simulink model "A14_Servoachse_Kaskade"  (R2017b)
settings: Solver=ode45  StartTime=0.0  StopTime=10  FixedStep=0.001  MaxStep=1e-4  RelTol=1e-3  EnableMultiTasking=on
values from neighbouring files (symbols this model uses):
  CD = 1e1    (= 10)    [A14_Konstanten.m]    (also in A17_Konstanten.m = 100; A8_Konstanten.m = 20; A9_Konstanten.m = 0.1)
  CF = 1e4    (= 10000)    [A13_Konstanten.m]    (also in A14_Konstanten.m; A17_Konstanten.m = 50000; A8_Konstanten.m = 10000000; A9_Konstanten.m)
  CM = 7.1e-7    (= 7.1e-07)    [A10_Konstanten.m]    (also in A13_Konstanten.m; A14_Konstanten.m; A16_Konstanten.m)
  CR = 0.2    [A13_Konstanten.m]    (also in A14_Konstanten.m; A17_Konstanten.m = 100; A9_Konstanten.m = 1; Z_Parametrisierung_Skript.m = [0.5,1,5])
  FReib = 0.5    [A13_Konstanten.m]    (also in A14_Konstanten.m)
  Imax = 4.81    [A10_Konstanten.m]    (also in A13_Konstanten.m; A14_Konstanten.m; A16_Konstanten.m)
  JM = JR + JG    (= 1.38e-06)    [A13_Konstanten.m]    (also in A14_Konstanten.m)
  KM = 38.4e-3    (= 0.0384)    [A10_Konstanten.m]    (also in A13_Konstanten.m; A14_Konstanten.m; A16_Konstanten.m)
  KN = 1/(2*pi*KM)    (= 4.14465997635)    [A10_Konstanten.m]    (also in A13_Konstanten.m; A14_Konstanten.m; A16_Konstanten.m)
  LA = 4.64e-4    (= 0.000464)    [A10_Konstanten.m]    (also in A13_Konstanten.m; A14_Konstanten.m; A16_Konstanten.m)
  m1 = 1    [A13_Konstanten.m]    (also in A14_Konstanten.m; A17_Konstanten.m = 4; A8_Konstanten.m = 20)
  nmax = 99    [A10_Konstanten.m]    (also in A13_Konstanten.m; A14_Konstanten.m; A16_Konstanten.m)
  R = 0.02    [A10_Konstanten.m]    (also in A13_Konstanten.m = 0.04; A14_Konstanten.m = 0.04; A16_Konstanten.m)
  RA = 4.99    [A10_Konstanten.m]    (also in A13_Konstanten.m; A14_Konstanten.m; A16_Konstanten.m)
  Ti = Ue/(2*pi*R)    (= 15.9154943092)    [A14_Konstanten.m]
  Tisens = 2e-5    (= 2e-05)    [A14_Konstanten.m]
  Tnsens = 8e-5    (= 8e-05)    [A14_Konstanten.m]
  TPWM = 2e-5    (= 2e-05)    [A14_Konstanten.m]
  Tssens = Tnsens    (= 8e-05)    [A14_Konstanten.m]
  TVn = 4*(2*(TPWM+Tisens)+Tnsens)    (= 0.00064)    [A14_Konstanten.m]
  Ue = 4    [A13_Konstanten.m]    (also in A14_Konstanten.m)
  Umax = 24    [A10_Konstanten.m]    (also in A13_Konstanten.m; A14_Konstanten.m; A16_Konstanten.m; A17_Konstanten.m = 120)
  WGrad = 0.85    [A13_Konstanten.m]    (also in A14_Konstanten.m)
undefined symbols (not defined in the file or in its folder): sigbuilder_block
libraries: simulink x4
settings Model: Creator=jbaur  LastModifiedBy=jbaur
settings DataIOCC: ExternalInput=X1  SaveFormat=StructureWithTime  InspectSignalLogs=on  SignalLoggingName=sigsOut
settings OptimizationCC: DefaultParameterBehavior=Inlined  InlineInvariantSignals=on  BufferReuse=off  ExpressionDepthLimit=2147483647  InitFltsAndDblsToZero=on  LifeSpan=inf
settings DebuggingCC: SaveWithParameterizedLinksMsg=none  SignalResolutionControl=TryResolveAllWithWarning  MultiTaskDSMMsg=warning  MultiTaskCondExecSysMsg=none  StateNameClashWarn=warning  InitInArrayFormatMsg=none  SFUnexpectedBacktrackingDiag=warning  SFNoUnconditionalDefaultTransitionDiag=warning  SFExecutionAtInitializationDiag=none
settings HardwareCC: ProdBitPerPointer=32  ProdBitPerSizeT=32  ProdBitPerPtrDiffT=32  ProdLargestAtomicFloat=None  ProdIntDivRoundTo=Undefined  ProdEndianess=Unspecified  ProdWordSize=32  ProdHWDeviceType=32-bit Generic  TargetBitPerPointer=64  TargetBitPerSizeT=64  TargetBitPerPtrDiffT=64  TargetLongLongMode=on  TargetIntDivRoundTo=Zero  TargetEndianess=LittleEndian  TargetWordSize=64  TargetHWDeviceType=MATLAB Host  ProdEqTarget=off
settings ModelReferenceCC: PropagateSignalLabelsOutOfModel=off
settings CodeAppCC: StateflowObjectComments=on
settings GRTTargetCC: TargetFcnLib=ansi_tfl_tmw.mat  TargetLangStandard=C89/C90 (ANSI)  ModelReferenceCompliant=off  GeneratePreprocessorConditionals=Disable all  CombineOutputUpdateFcns=off  MatFileLogging=off  GRTInterface=on
settings ConfigComp: CovMetricSettings=dw  CovHtmlReporting=on  CovSaveCumulativeToWorkspaceVar=on  CovSaveSingleToWorkspaceVar=on  CovExternalEMLEnable=off  CovSFcnEnable=off

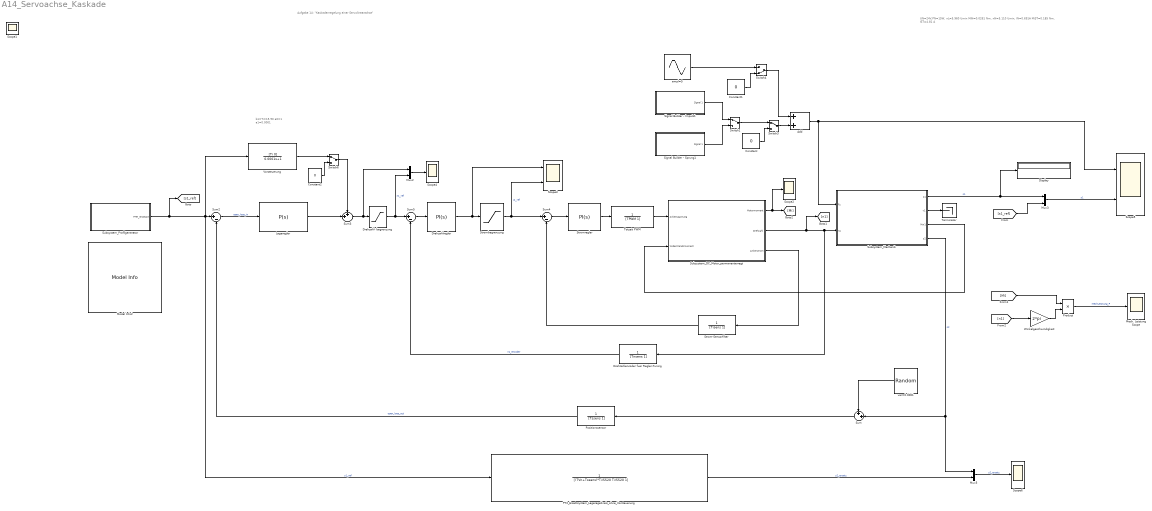
== system A14_Servoachse_Kaskade ==
  note: b1=Ti=15.90
      | a0=1
      | a1=0.0001
  note: Aufgabe 14: "Kaskadenregelung einer Servolinearachse"
  note: UN=24V,PN=15W, nL=5.960 Umin
      | MiN=0.0261 Nm, nN=5.110 Umin, IN=0.691A
      | MiST=0.185 Nm, IST=4.81 A
  Add : Sum
  Constant : Constant  Value=0
  Constant1 : Constant  Value=0
  Constant2 : Constant  Value=0
  Display : Display
  Drehzahl- begrenzung : Saturate  UpperLimit=nmax  LowerLimit=-nmax
  Drehzahlencoder fuer Regler-Tuning : TransferFcn  Denominator=[Tnsens 1]
  Drehzahlregler : simulink/Continuous/PID Controller  Controller=PI  TimeDomain=Continuous-time  SampleTime=-1  IntegratorMethod=Forward Euler  FilterMethod=Forward Euler  Form=Ideal  UseFilter=on  ControllerParametersSource=internal  P=1  I=1  D=0  N=1000  InitialConditionSource=internal  InitialConditionForIntegrator=0  InitialConditionForFilter=0  ExternalReset=none  LimitOutput=on  UpperSaturationLimit=Imax  LowerSaturationLimit=-Imax  LinearizeAsGain=off  AntiWindupMode=clamping  Kb=1  TrackingMode=off  Kt=1  PParamMin=[]  PParamMax=[]  IParamMin=[]  IParamMax=[]  DParamMin=[]  DParamMax=[]  NParamMin=[]  NParamMax=[]  KbParamMin=[]  KbParamMax=[]  KtParamMin=[]  KtParamMax=[]  POutMin=[]  POutMax=[]  IOutMin=[]  IOutMax=[]  DOutMin=[]  DOutMax=[]  NOutMin=[]  NOutMax=[]  KbOutMin=[]  KbOutMax=[]  KtOutMin=[]  KtOutMax=[]  IntegratorOutMin=[]  IntegratorOutMax=[]  FilterOutMin=[]  FilterOutMax=[]  SumOutMin=[]  SumOutMax=[]  SumI1OutMin=[]  SumI1OutMax=[]  SumI2OutMin=[]  SumI2OutMax=[]  SumI3OutMin=[]  SumI3OutMax=[]  SumDOutMin=[]  SumDOutMax=[]  SaturationOutMin=[]  SaturationOutMax=[]  IntegratorContinuousStateAttributes=''  IntegratorStateMustResolveToSignalObject=off  IntegratorRTWStateStorageClass=Auto  FilterContinuousStateAttributes=''  FilterStateMustResolveToSignalObject=off  FilterRTWStateStorageClass=Auto  DifferentiatorICPrevScaledInput=0  DifferentiatorOutMin=[]  DifferentiatorOutMax=[]  InitialConditionSetting=State (most efficient)  FilterDiffOutCoefMin=[]  FilterDiffOutCoefMax=[]  SumDenOutMin=[]  SumDenOutMax=[]  SumNumOutMin=[]  SumNumOutMax=[]  ReciprocalOutMin=[]  ReciprocalOutMax=[]  DivideOutMin=[]  DivideOutMax=[]  TunerSelectOption=Transfer Function Based (PID Tuner App)
  Lageregler : simulink/Continuous/PID Controller  Controller=P  TimeDomain=Continuous-time  SampleTime=-1  IntegratorMethod=Forward Euler  FilterMethod=Forward Euler  Form=Ideal  UseFilter=on  ControllerParametersSource=internal  P=1  I=2096.01243911413  D=0  N=100  InitialConditionSource=internal  InitialConditionForIntegrator=0  InitialConditionForFilter=0  ExternalReset=none  LimitOutput=off  UpperSaturationLimit=nmax  LowerSaturationLimit=-nmax  LinearizeAsGain=off  AntiWindupMode=none  Kb=1  TrackingMode=off  Kt=1  PParamMin=[]  PParamMax=[]  IParamMin=[]  IParamMax=[]  DParamMin=[]  DParamMax=[]  NParamMin=[]  NParamMax=[]  KbParamMin=[]  KbParamMax=[]  KtParamMin=[]  KtParamMax=[]  POutMin=[]  POutMax=[]  IOutMin=[]  IOutMax=[]  DOutMin=[]  DOutMax=[]  NOutMin=[]  NOutMax=[]  KbOutMin=[]  KbOutMax=[]  KtOutMin=[]  KtOutMax=[]  IntegratorOutMin=[]  IntegratorOutMax=[]  FilterOutMin=[]  FilterOutMax=[]  SumOutMin=[]  SumOutMax=[]  SumI1OutMin=[]  SumI1OutMax=[]  SumI2OutMin=[]  SumI2OutMax=[]  SumI3OutMin=[]  SumI3OutMax=[]  SumDOutMin=[]  SumDOutMax=[]  SaturationOutMin=[]  SaturationOutMax=[]  IntegratorContinuousStateAttributes=''  IntegratorStateMustResolveToSignalObject=off  IntegratorRTWStateStorageClass=Auto  FilterContinuousStateAttributes=''  FilterStateMustResolveToSignalObject=off  FilterRTWStateStorageClass=Auto  DifferentiatorICPrevScaledInput=0  DifferentiatorOutMin=[]  DifferentiatorOutMax=[]  InitialConditionSetting=State (most efficient)  FilterDiffOutCoefMin=[]  FilterDiffOutCoefMax=[]  SumDenOutMin=[]  SumDenOutMax=[]  SumNumOutMin=[]  SumNumOutMax=[]  ReciprocalOutMin=[]  ReciprocalOutMax=[]  DivideOutMin=[]  DivideOutMax=[]  TunerSelectOption=Transfer Function Based (PID Tuner App)
  Mech. Leistung Scope : Scope
  Model Info2 : simulink/Model-Wide Utilities/Model Info  Frame=on  DisplayStringWithTags=|  HorizontalTextAlignment=Left  LeftAlignmentValue=0.02
      | Bewegungsprofil:
      | ------------------------
      | Tmax = 1s
      | smax = 0,5m
      | vmax = 1 m/s
      | amax = 2 m/s^2
  Mux2 : Mux  Inputs=2
  Mux3 : Mux  Inputs=2
  Mux5 : Mux  Inputs=2
  PT2_Ersatzsystem_Lageregelkreis_ohne_Vorsteuerung : TransferFcn  Denominator=[(TVn+Tssens)*Ti/5520 Ti/5520 1]
  "Positionssensor " : TransferFcn  Denominator=[Tssens 1]
  Product : Product  RndMeth=Zero
  Scope{1..2,4,6} (4 alike) : Scope
  Scope3 : Scope  NumInputPorts=2
  Scope5 : Scope  NumInputPorts=2
  Signal Builder - Impuls1 : Subsystem  Tag=STV Subsys  LoadFcn=sigbuilder_block('load');  StartFcn=sigbuilder_block('start');  StopFcn=sigbuilder_block('stop');  ClipboardFcn=sigbuilder_block('clipboard');  mask(Sigbuilder block){tuvar=[0:10]}
      mask help: Simulink:masks:SigbuilderBlock_MD
      mask init:
      | if ~strcmp(get_param(bdroot(gcbh),'SimulationStatus'),'stopped') tuvar = sigbuilder_block('maskInit'); end
      settings: CopyFcn=sigbuilder_block('copy');  DeleteFcn=sigbuilder_block('delete');  ModelCloseFcn=sigbuilder_block('modelClose');  PreSaveFcn=sigbuilder_block('preSave');  PauseFcn=sigbuilder_block('pause');  ContinueFcn=sigbuilder_block('continue');  NameChangeFcn=sigbuilder_block('namechange');  OpenFcn=sigbuilder_block('open',[431.25 106.5 550.5 399.75 ]);  CloseFcn=sigbuilder_block('close');
      mask Display: plot(0, 0, 100, 100,[2, 2, 32, 32, 2], [68, 8, 8, 68, 68],[32, 2], [38, 38], [32, 19, 2],[53, 60, 44], [32, 17, 17, 2],[16, 16, 31, 31]);txt = getActiveGroup(gcbh);text(2, 100, txt,'verticalAlignment', 'top');
  Signal Builder - Sprung1 : Subsystem  Tag=STV Subsys  LoadFcn=sigbuilder_block('load');  StartFcn=sigbuilder_block('start');  StopFcn=sigbuilder_block('stop');  ClipboardFcn=sigbuilder_block('clipboard');  mask(Sigbuilder block){tuvar=[0:10]}
      mask help: Simulink:masks:SigbuilderBlock_MD
      mask init:
      | if ~strcmp(get_param(bdroot(gcbh),'SimulationStatus'),'stopped') tuvar = sigbuilder_block('maskInit'); end
      settings: CopyFcn=sigbuilder_block('copy');  DeleteFcn=sigbuilder_block('delete');  ModelCloseFcn=sigbuilder_block('modelClose');  PreSaveFcn=sigbuilder_block('preSave');  PauseFcn=sigbuilder_block('pause');  ContinueFcn=sigbuilder_block('continue');  NameChangeFcn=sigbuilder_block('namechange');  OpenFcn=sigbuilder_block('open',[1699.5 180.75 550.5 399.75 ]);  CloseFcn=sigbuilder_block('close');
      mask Display: plot(0, 0, 100, 100,[2, 2, 32, 32, 2], [68, 8, 8, 68, 68],[32, 2], [38, 38], [32, 19, 2],[53, 60, 44], [32, 17, 17, 2],[16, 16, 31, 31]);txt = getActiveGroup(gcbh);text(2, 100, txt,'verticalAlignment', 'top');
  Strom-Sensorfilter : TransferFcn  Denominator=[Tisens 1]
  Strombegrenzung : Saturate  UpperLimit=Imax  LowerLimit=-Imax
  Stromregler : simulink/Continuous/PID Controller  Controller=PI  TimeDomain=Continuous-time  SampleTime=-1  IntegratorMethod=Forward Euler  FilterMethod=Forward Euler  Form=Ideal  UseFilter=on  ControllerParametersSource=internal  P=1  I=1  D=-0.00136816077946148  N=3731.68343054543  InitialConditionSource=internal  InitialConditionForIntegrator=0  InitialConditionForFilter=0  ExternalReset=none  LimitOutput=off  UpperSaturationLimit=Umax  LowerSaturationLimit=-Umax  LinearizeAsGain=on  AntiWindupMode=clamping  Kb=1  TrackingMode=off  Kt=1  PParamMin=[]  PParamMax=[]  IParamMin=[]  IParamMax=[]  DParamMin=[]  DParamMax=[]  NParamMin=[]  NParamMax=[]  KbParamMin=[]  KbParamMax=[]  KtParamMin=[]  KtParamMax=[]  POutMin=[]  POutMax=[]  IOutMin=[]  IOutMax=[]  DOutMin=[]  DOutMax=[]  NOutMin=[]  NOutMax=[]  KbOutMin=[]  KbOutMax=[]  KtOutMin=[]  KtOutMax=[]  IntegratorOutMin=[]  IntegratorOutMax=[]  FilterOutMin=[]  FilterOutMax=[]  SumOutMin=[]  SumOutMax=[]  SumI1OutMin=[]  SumI1OutMax=[]  SumI2OutMin=[]  SumI2OutMax=[]  SumI3OutMin=[]  SumI3OutMax=[]  SumDOutMin=[]  SumDOutMax=[]  SaturationOutMin=[]  SaturationOutMax=[]  IntegratorContinuousStateAttributes=''  IntegratorStateMustResolveToSignalObject=off  IntegratorRTWStateStorageClass=Auto  FilterContinuousStateAttributes=''  FilterStateMustResolveToSignalObject=off  FilterRTWStateStorageClass=Auto  DifferentiatorICPrevScaledInput=0  DifferentiatorOutMin=[]  DifferentiatorOutMax=[]  InitialConditionSetting=State (most efficient)  FilterDiffOutCoefMin=[]  FilterDiffOutCoefMax=[]  SumDenOutMin=[]  SumDenOutMax=[]  SumNumOutMin=[]  SumNumOutMax=[]  ReciprocalOutMin=[]  ReciprocalOutMax=[]  DivideOutMin=[]  DivideOutMax=[]  TunerSelectOption=Transfer Function Based (PID Tuner App)
  Subsystem_DC_Motor_permanenterregt : Subsystem
  Subsystem_Mechanik : Subsystem
  Subsystem_Profilgenerator : Subsystem
  Sum : Sum  Inputs=++|
  Sum2 : Sum  Inputs=|+-  SaturateOnIntegerOverflow=on
  Sum3 : Sum  Inputs=++|  SaturateOnIntegerOverflow=on
  Sum4 : Sum  Inputs=|+-
  Sum5 : Sum  Inputs=|+-  SaturateOnIntegerOverflow=on
  Switch1 : ManualSwitch
  Switch3 : ManualSwitch
  Switch4 : ManualSwitch  CurrentSetting=0
  Switch6 : ManualSwitch
  Terminator : Terminator
  Totzeit PWM : TransferFcn  Denominator=[TPWM 1]
  Vorsteuerung : TransferFcn  Numerator=[Ti 0]  Denominator=[0.0001 1]
  Winkelgeschwindigkeit : Gain  Gain=2*pi
  ampl=5 : Sin  Amplitude=5  Frequency=2*pi*20  SampleTime=0
  var=0.0001 : RandomNumber  Variance=0  SampleTime=0.001
  wires:
  Sum5/1 -> Drehzahlregler/1
  Sum4/1 -> Stromregler/1
  Stromregler/1 -> Totzeit PWM/1
  Drehzahlregler/1 -> Strombegrenzung/1, Scope3/1
  Strombegrenzung/1 -> Sum4/1, Scope3/2  "iA_ref"
  Sum2/1 -> Lageregler/1  "open_loop_in"
  Subsystem_Profilgenerator/1(FHR_Groesse) -> PT2_Ersatzsystem_Lageregelkreis_ohne_Vorsteuerung/1, Sum2/1, Vorsteuerung/1, [s1_ref]  "s1_ref"
  Lageregler/1 -> Sum3/2
  Sum3/1 -> Mux2/1, Drehzahl- begrenzung/1
  Mux2/1 -> Scope4/1
  Product/1 -> Mech. Leistung Scope/1  "MechLeistung_P"
  [Mi] -> Product/1
  [n1] -> Winkelgeschwindigkeit/1
  Winkelgeschwindigkeit/1 -> Product/2
  Subsystem_Mechanik/2(v1) -> Terminator/1
  Strom-Sensorfilter/1 -> Sum4/2
  Totzeit PWM/1 -> Subsystem_DC_Motor_permanenterregt/1(Ankerspannung)
  Subsystem_Mechanik/1(s1) -> Display/1, Mux3/1  "s1"
  [s1_ref] -> Mux3/2
  Mux3/1 -> Scope5/2  "s1"
  Mux5/1 -> Scope6/1  "s2_ersatz"
  Signal Builder - Impuls1/1(Signal 1) -> Switch1/1
  Signal Builder - Sprung1/1(Signal 1) -> Switch1/2
  Drehzahlencoder fuer Regler-Tuning/1 -> Sum5/2  "n1_encoder"
  var=0.0001/1 -> Sum/1
  Add/1 -> Subsystem_Mechanik/1(Fz), Scope5/1
  Switch3/1 -> Add/2
  Switch1/1 -> Switch3/1
  Constant/1 -> Switch3/2
  Drehzahl- begrenzung/1 -> Sum5/1, Mux2/2  "n1_ref"
  Subsystem_DC_Motor_permanenterregt/2(Drehzahl) -> [n1], Drehzahlencoder fuer Regler-Tuning/1, Subsystem_Mechanik/2(n1)
  PT2_Ersatzsystem_Lageregelkreis_ohne_Vorsteuerung/1 -> Mux5/2  "s2_ersatz"
  "Positionssensor "/1 -> Sum2/2  "open_loop_out"
  Switch4/1 -> Add/1
  Constant1/1 -> Switch4/2
  ampl=5/1 -> Switch4/1
  Switch6/1 -> Sum3/1
  Constant2/1 -> Switch6/2
  Vorsteuerung/1 -> Switch6/1
  Sum/1 -> "Positionssensor "/1
  Subsystem_Mechanik/3(Mw1) -> Subsystem_DC_Motor_permanenterregt/2(Widerstandsmoment)
  Subsystem_Mechanik/4(s2) -> Mux5/1, Sum/2  "s2"
  Subsystem_DC_Motor_permanenterregt/1(Motormoment) -> Scope2/1, [Mi]
  Subsystem_DC_Motor_permanenterregt/3(Ankerstrom) -> Strom-Sensorfilter/1

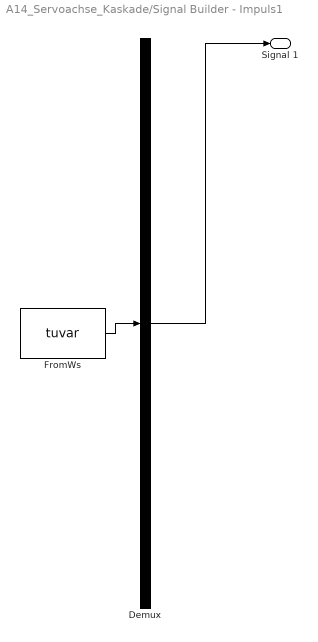
== system A14_Servoachse_Kaskade/Signal Builder - Impuls1 ==
  Demux : Demux  Tag=STV Demux  Outputs=1
  FromWs : FromWorkspace  Tag=STV FromWs  VariableName=tuvar  SampleTime=0
      SigBuilderData=|
      | common.afterFinalStr = 'Extrapolate'
      | common.sampleTime = 0
      | dataSet.timeRange = [0 20]
      | dataSet.name = 'Group 1'
      | sbobj.Groups.Name = 'Group 1'
      | sbobj.Groups.Signals.Name = 'Signal 1'
      | sbobj.Groups.Signals.XData = [0 5 5 7 7 20]
      | sbobj.Groups.Signals.YData = [0 0 10 10 0 0]
      | sbobj.Groups.TimeRange = [0 20]
  Signal 1 : Outport  Tag=STV Outport
  wires:
  Demux/1 -> Signal 1/1
  FromWs/1 -> Demux/1

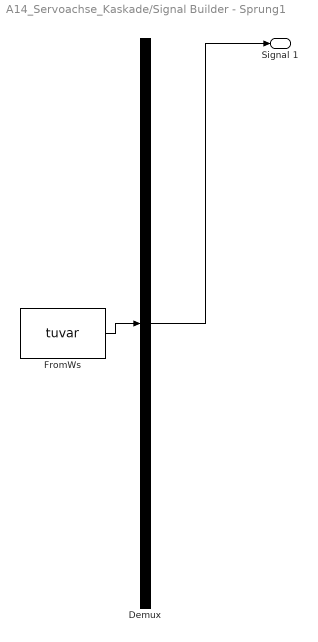
== system A14_Servoachse_Kaskade/Signal Builder - Sprung1 ==
  Demux : Demux  Tag=STV Demux  Outputs=1
  FromWs : FromWorkspace  Tag=STV FromWs  VariableName=tuvar  SampleTime=0
      SigBuilderData=|
      | common.afterFinalStr = 'Extrapolate'
      | common.sampleTime = 0
      | dataSet.timeRange = [0 20]
      | dataSet.name = 'Group 1'
      | sbobj.Groups.Name = 'Group 1'
      | sbobj.Groups.Signals.Name = 'Signal 1'
      | sbobj.Groups.Signals.XData = [0 5 5 20]
      | sbobj.Groups.Signals.YData = [0 0 10 10]
      | sbobj.Groups.TimeRange = [0 20]
  Signal 1 : Outport  Tag=STV Outport
  wires:
  Demux/1 -> Signal 1/1
  FromWs/1 -> Demux/1

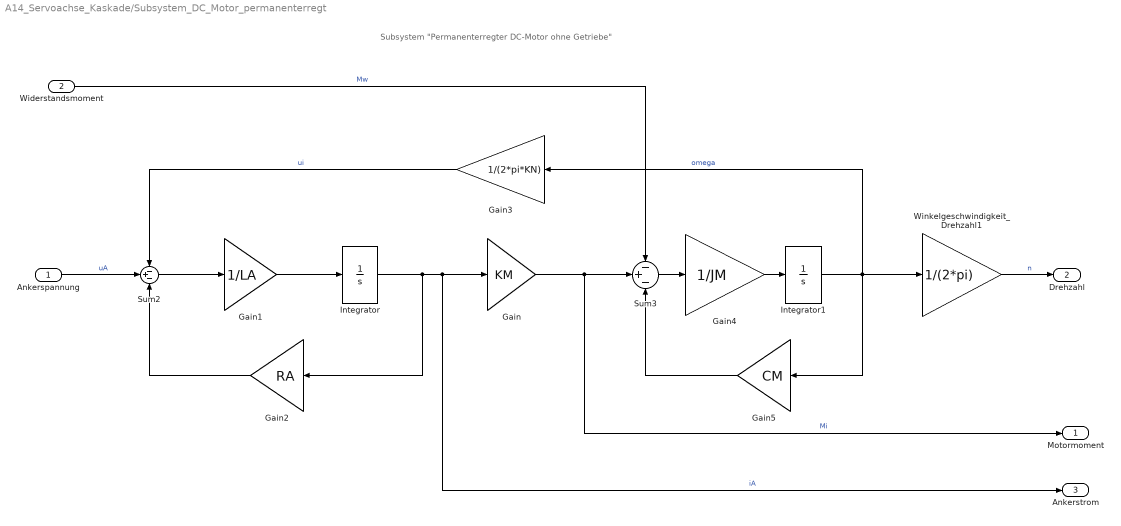
== system A14_Servoachse_Kaskade/Subsystem_DC_Motor_permanenterregt ==
  note: Subsystem "Permanenterregter DC-Motor ohne Getriebe"
  Ankerspannung : Inport
  Widerstandsmoment : Inport  Port=2
  Gain : Gain  Gain=KM
  Gain1 : Gain  Gain=1/LA
  Gain2 : Gain  Gain=RA
  Gain3 : Gain  Gain=1/(2*pi*KN)
  Gain4 : Gain  Gain=1/JM
  Gain5 : Gain  Gain=CM
  Integrator : Integrator
  Integrator1 : Integrator
  Sum2 : Sum  Inputs=-+-
  Sum3 : Sum  Inputs=-+-
  Winkelgeschwindigkeit_Drehzahl1 : Gain  Gain=1/(2*pi)
  Motormoment : Outport
  Drehzahl : Outport  Port=2
  Ankerstrom : Outport  Port=3
  wires:
  Ankerspannung/1 -> Sum2/2  "uA"
  Gain3/1 -> Sum2/1  "ui"
  Gain/1 -> Sum3/2, Motormoment/1  "Mi"
  Winkelgeschwindigkeit_Drehzahl1/1 -> Drehzahl/1  "n"
  Sum2/1 -> Gain1/1
  Gain1/1 -> Integrator/1
  Integrator/1 -> Gain2/1, Ankerstrom/1, Gain/1  "iA"
  Sum3/1 -> Gain4/1
  Gain4/1 -> Integrator1/1
  Integrator1/1 -> Gain3/1, Winkelgeschwindigkeit_Drehzahl1/1, Gain5/1  "omega"
  Gain5/1 -> Sum3/3
  Gain2/1 -> Sum2/3
  Widerstandsmoment/1 -> Sum3/1  "Mw"

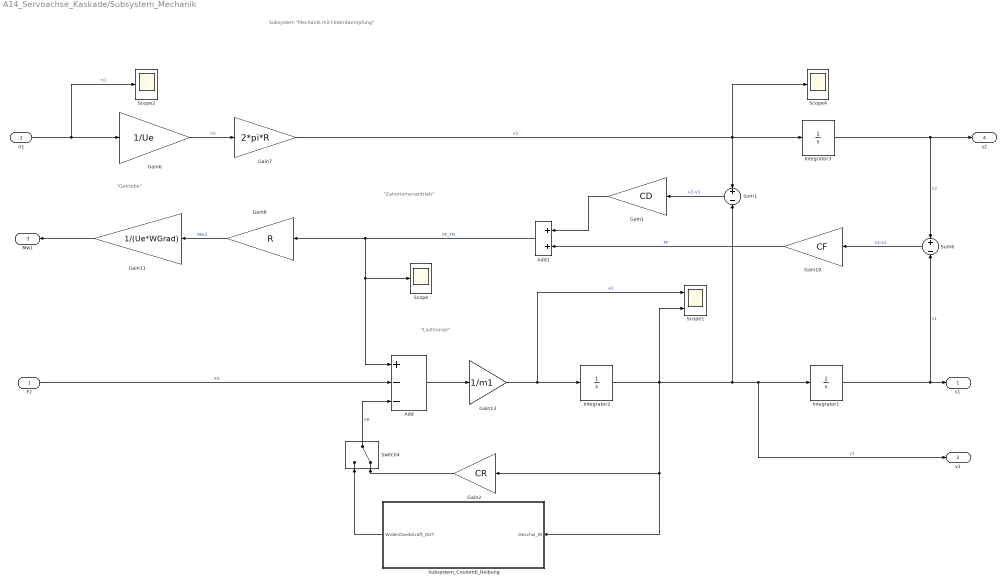
== system A14_Servoachse_Kaskade/Subsystem_Mechanik ==
  note: Subsystem "Mechanik mit Federdaempfung"
  note: "Lastmasse"
  note: "Zahnriemenantrieb"
  note: "Getriebe"
  Fz : Inport
  n1 : Inport  Port=2
  Add : Sum  Inputs=+--
  Add1 : Sum
  Gain1 : Gain  Gain=CD
  Gain10 : Gain  Gain=CF
  Gain11 : Gain  Gain=1/(Ue*WGrad)
  Gain13 : Gain  Gain=1/m1
  Gain2 : Gain  Gain=CR
  Gain6 : Gain  Gain=1/Ue
  Gain7 : Gain  Gain=2*pi*R
  Gain8 : Gain  Gain=R
  Integrator1 : Integrator
  Integrator2 : Integrator
  Integrator3 : Integrator
  Scope : Scope
  Scope1 : Scope  NumInputPorts=2
  Scope2 : Scope
  Scope4 : Scope
  Subsystem_Coulomb_Reibung : Subsystem
  Sum1 : Sum  Inputs=+|-
  Sum6 : Sum  Inputs=+|-
  Switch4 : ManualSwitch  CurrentSetting=0
  s1 : Outport
  v1 : Outport  Port=2
  Mw1 : Outport  Port=3
  s2 : Outport  Port=4
  wires:
  Integrator1/1 -> s1/1, Sum6/2  "s1"
  Add/1 -> Gain13/1
  Gain13/1 -> Scope1/1, Integrator2/1  "a1"
  Gain7/1 -> Integrator3/1, Scope4/1, Sum1/1  "v2"
  Gain8/1 -> Gain11/1  "Mw2"
  Sum6/1 -> Gain10/1  "s2-s1"
  n1/1 -> Scope2/1, Gain6/1  "n1"
  Gain6/1 -> Gain7/1  "n2"
  Fz/1 -> Add/2  "FZ"
  Gain11/1 -> Mw1/1
  Sum1/1 -> Gain1/1  "v2-v1"
  Gain10/1 -> Add1/2  "FF"
  Gain1/1 -> Add1/1
  Add1/1 -> Scope/1, Add/1, Gain8/1  "FF_FD"
  Integrator3/1 -> s2/1, Sum6/1  "s2"
  Integrator2/1 -> Subsystem_Coulomb_Reibung/1(Geschw_IN), Gain2/1, Scope1/2, Sum1/2, v1/1, Integrator1/1  "v1"
  Switch4/1 -> Add/3  "FR"
  Gain2/1 -> Switch4/2
  Subsystem_Coulomb_Reibung/1(Widerstandskraft_OUT) -> Switch4/1

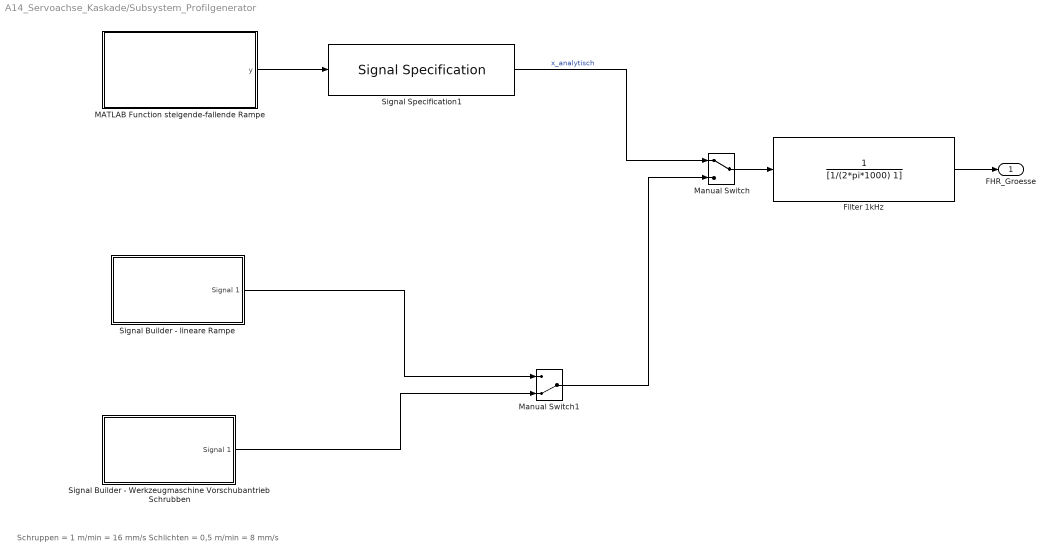
== system A14_Servoachse_Kaskade/Subsystem_Profilgenerator ==
  note: Schruppen = 1 m/min = 16 mm/s
      | Schlichten = 0,5 m/min = 8 mm/s
  Filter 1kHz : TransferFcn  Denominator=[1/(2*pi*1000) 1]
  MATLAB Function steigende-fallende Rampe : MATLAB Function  TreatAsAtomicUnit=on
  Manual Switch : ManualSwitch  SampleTime=1e-4
  Manual Switch1 : ManualSwitch  CurrentSetting=0  SampleTime=1e-4
  Signal Builder - Werkzeugmaschine Vorschubantrieb Schrubben : Subsystem  Tag=STV Subsys  LoadFcn=sigbuilder_block('load');  StartFcn=sigbuilder_block('start');  StopFcn=sigbuilder_block('stop');  ClipboardFcn=sigbuilder_block('clipboard');  mask(Sigbuilder block){tuvar=[0:10]}
      mask help: Create and generate interchangeable groups of signals whose waveforms are piecewise linear.
      mask init:
      | if ~strcmp(get_param(bdroot(gcbh),'SimulationStatus'),'stopped') tuvar = sigbuilder_block('maskInit'); end
      settings: CopyFcn=sigbuilder_block('copy');  DeleteFcn=sigbuilder_block('delete');  ModelCloseFcn=sigbuilder_block('modelClose');  PreSaveFcn=sigbuilder_block('preSave');  PauseFcn=sigbuilder_block('pause')  ContinueFcn=sigbuilder_block('continue')  NameChangeFcn=sigbuilder_block('namechange');  OpenFcn=sigbuilder_block('open',[437.25 199.5 550.5 399.75 ]);  CloseFcn=sigbuilder_block('close');
      mask Display: plot(0, 0, 100, 100,[2, 2, 32, 32, 2], [68, 8, 8, 68, 68],[32, 2], [38, 38], [32, 19, 2],[53, 60, 44], [32, 17, 17, 2],[16, 16, 31, 31]);txt = getActiveGroup(gcbh);text(2, 100, txt,'verticalAlignment', 'top');
  Signal Builder - lineare Rampe : Subsystem  Tag=STV Subsys  LoadFcn=sigbuilder_block('load');  StartFcn=sigbuilder_block('start');  StopFcn=sigbuilder_block('stop');  ClipboardFcn=sigbuilder_block('clipboard');  mask(Sigbuilder block){tuvar=[0:10]}
      mask help: Create and generate interchangeable groups of signals whose waveforms are piecewise linear.
      mask init:
      | if ~strcmp(get_param(bdroot(gcbh),'SimulationStatus'),'stopped') tuvar = sigbuilder_block('maskInit'); end
      settings: CopyFcn=sigbuilder_block('copy');  DeleteFcn=sigbuilder_block('delete');  ModelCloseFcn=sigbuilder_block('modelClose');  PreSaveFcn=sigbuilder_block('preSave');  PauseFcn=sigbuilder_block('pause')  ContinueFcn=sigbuilder_block('continue')  NameChangeFcn=sigbuilder_block('namechange');  OpenFcn=sigbuilder_block('open',[437.25 199.5 550.5 399.75 ]);  CloseFcn=sigbuilder_block('close');
      mask Display: plot(0, 0, 100, 100,[2, 2, 32, 32, 2], [68, 8, 8, 68, 68],[32, 2], [38, 38], [32, 19, 2],[53, 60, 44], [32, 17, 17, 2],[16, 16, 31, 31]);txt = getActiveGroup(gcbh);text(2, 100, txt,'verticalAlignment', 'top');
  Signal Specification1 : SignalSpecification  SampleTime=1e-4
  FHR_Groesse : Outport
  wires:
  MATLAB Function steigende-fallende Rampe/1(y) -> Signal Specification1/1
  Manual Switch/1 -> Filter 1kHz/1
  Signal Specification1/1 -> Manual Switch/1  "x_analytisch"
  Filter 1kHz/1 -> FHR_Groesse/1
  Manual Switch1/1 -> Manual Switch/2
  Signal Builder - lineare Rampe/1(Signal 1) -> Manual Switch1/1
  Signal Builder - Werkzeugmaschine Vorschubantrieb Schrubben/1(Signal 1) -> Manual Switch1/2

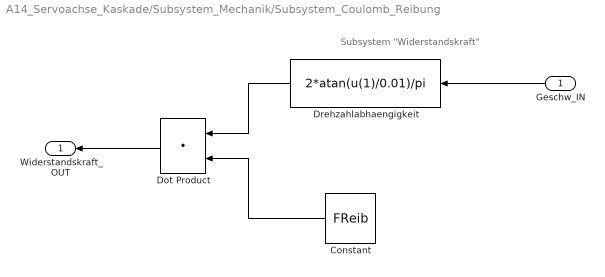
== system A14_Servoachse_Kaskade/Subsystem_Mechanik/Subsystem_Coulomb_Reibung ==
  note: Subsystem "Widerstandskraft"
  Geschw_IN : Inport
  Constant : Constant  Value=FReib
  Dot Product : DotProduct  InputSameDT=on  OutDataTypeStr=Inherit: Inherit via internal rule
  Drehzahlabhaengigkeit : Fcn  Expr=2*atan(u(1)/0.01)/pi
  Widerstandskraft_OUT : Outport
  wires:
  Constant/1 -> Dot Product/2
  Drehzahlabhaengigkeit/1 -> Dot Product/1
  Geschw_IN/1 -> Drehzahlabhaengigkeit/1
  Dot Product/1 -> Widerstandskraft_OUT/1

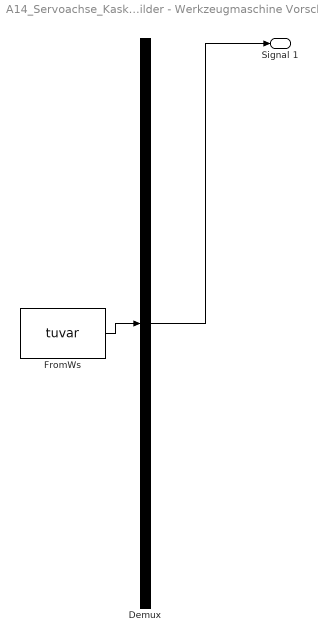
== system A14_Servoachse_Kaskade/Subsystem_Profilgenerator/Signal Builder - Werkzeugmaschine Vorschubantrieb Schrubben ==
  Demux : Demux  Tag=STV Demux  Outputs=1
  FromWs : FromWorkspace  Tag=STV FromWs  VariableName=tuvar  SampleTime=0
      SigBuilderData=|
      | common.afterFinalStr = 'Extrapolate'
      | common.sampleTime = 0
      | dataSet.timeRange = [0 10]
      | dataSet.name = 'Group 1'
      | sbobj.Groups.Name = 'Group 1'
      | sbobj.Groups.Signals.Name = 'Signal 1'
      | sbobj.Groups.Signals.XData = [0 6 10]
      | sbobj.Groups.Signals.YData = [0 0.1 0.1]
  Signal 1 : Outport  Tag=STV Outport
  wires:
  Demux/1 -> Signal 1/1
  FromWs/1 -> Demux/1

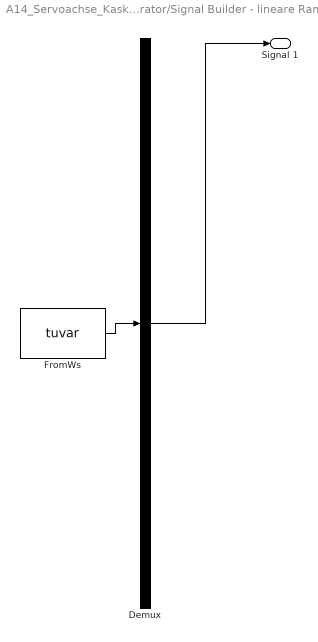
== system A14_Servoachse_Kaskade/Subsystem_Profilgenerator/Signal Builder - lineare Rampe ==
  Demux : Demux  Tag=STV Demux  Outputs=1
  FromWs : FromWorkspace  Tag=STV FromWs  VariableName=tuvar  SampleTime=0
      SigBuilderData=|
      | common.afterFinalStr = 'Extrapolate'
      | common.sampleTime = 0
      | dataSet.timeRange = [0 10]
      | dataSet.name = 'Group 1'
      | sbobj.Groups.Name = 'Group 1'
      | sbobj.Groups.Signals.Name = 'Signal 1'
      | sbobj.Groups.Signals.XData = [0 1 5 5 10]
      | sbobj.Groups.Signals.YData = [0 0.5 0.5 0 0]
  Signal 1 : Outport  Tag=STV Outport
  wires:
  Demux/1 -> Signal 1/1
  FromWs/1 -> Demux/1

== matlab function A14_Servoachse_Kaskade/Subsystem_Profilgenerator/MATLAB Function steigende-fallende Rampe ==
  data: y output
function y = Zeitfunktion

% Deklaration der persistenten (globalen) Zeitvariablen
Timestep = 1e-4;
persistent t

% Definition der Zeitfunktion
if isempty(t)
    t=0;
  else
    t = t + Timestep;
end

% Beschleunigungsbegrenztes Bewegungsprofil
T0 = 1;             % Startzeit Vorwärtsfahrt
T1 = 8;             % Startzeit Rückfahrt
s_max = 0.5;
T_max = 1;
t1 = T_max/2;
a_max = s_max/t1^2;
v_max = a_max*t1;

% Bereichsunterscheidung
if t<T0
    y = 0;
else
    if t<=T0+t1
        y = 0.5*a_max*(t-T0)^2;
    else
        if t <= T0+T_max
            y = 0.5*s_max + v_max*(t-t1-T0) - 0.5*a_max*(t-t1-T0)^2;
        else
            if t <= T1
                y = s_max;
            else
                if t <= T1+t1
                    y = s_max - 0.5*a_max*(t-T1)^2;
                else
                    if t <= T1+T_max
                        y = 0.5*s_max - v_max*(t-t1-T1) + 0.5*a_max*(t-t1-T1)^2;
                    else
                        y = 0;
                    end;
                end;
            end;
        end;
    end;
end;
